simulink model "Project2_1c_l_AbhayKela"  (R2014b)
settings: Solver=ode5  StartTime=0.0  StopTime=tf  FixedStep=0.01  RelTol=1e-3
values from neighbouring files (symbols this model uses):
  A = [1,4,2 ... (first row only)    [HW2.m]    (also in HW4_4.m = fx+(lambda1*g1)+(g1^2)+(lambda2*g2)+(g2^2); HW4_Problem4.m = f + lambda1*g1 + (g1^2) + lambda2*g2 + (g2^2); KelaAbhay_Project2.m = set_e')
  B = log(A)    [HW2.m]    (also in KelaAbhay_Project2.m = set_d')
  C = B(2,:)    [HW2.m]
  D = B(:,2).*A(:,1)    [HW2.m]
undefined symbols (not defined in the file or in its folder): xss
settings Model: Creator=axk7578  LastModifiedBy=axk7578

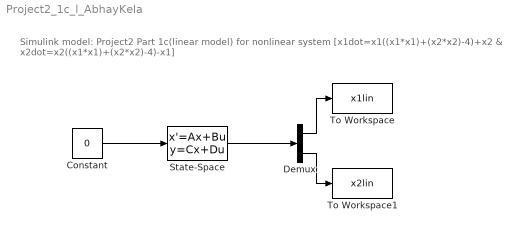
== system Project2_1c_l_AbhayKela ==
  note: Simulink model: Project2 Part 1c(linear model) for nonlinear system [x1dot=x1((x1*x1)+(x2*x2)-4)+x2 & x2dot=x2((x1*x1)+(x2*x2)-4)-x1]
  Constant : Constant  Value=0
  Demux : Demux  Outputs=2
  State-Space : StateSpace  A=A  B=B  C=C  D=D  X0=xss
  To Workspace : ToWorkspace  VariableName=x1lin  SampleTime=-1
  To Workspace1 : ToWorkspace  VariableName=x2lin  SampleTime=-1
  wires:
  State-Space/1 -> Demux/1
  Constant/1 -> State-Space/1
  Demux/1 -> To Workspace/1
  Demux/2 -> To Workspace1/1
